simulink model "sim_exp2"  (R2018a)
settings: Solver=VariableStepAuto  StartTime=0.0  StopTime=800  RelTol=1e-3
settings Model: Creator=Halil Temurtaş  LastModifiedBy=Halil Temurtaş

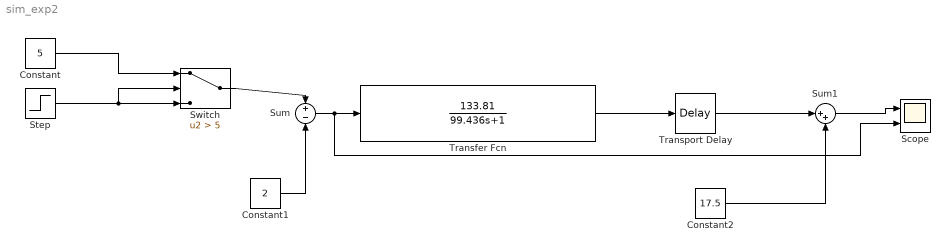
== system sim_exp2 ==
  Constant : Constant  Value=5
  Constant1 : Constant  Value=2
  Constant2 : Constant  Value=17.5
  Scope : Scope  NumInputPorts=2
  Step : Step  Time=0  Before=2  After=3.5  SampleTime=0
  Sum : Sum  Inputs=+-
  Sum1 : Sum  Inputs=|++
  Switch : Switch  Criteria=u2 > Threshold  Threshold=5
  Transfer Fcn : TransferFcn  Numerator=[133.81]  Denominator=[99.436 1]
  Transport Delay : TransportDelay  DelayTime=50.3
  wires:
  Step/1 -> Switch/3, Switch/2
  Constant/1 -> Switch/1
  Switch/1 -> Sum/1
  Constant1/1 -> Sum/2
  Sum/1 -> Scope/2, Transfer Fcn/1
  Transfer Fcn/1 -> Transport Delay/1
  Transport Delay/1 -> Sum1/1
  Constant2/1 -> Sum1/2
  Sum1/1 -> Scope/1
